simulink library "INT_InjSys_Co"  (R2016b)
settings: Solver=VariableStepAuto  StartTime=0.0  StopTime=10.0  RelTol=1e-3
settings Model: Creator=Administrator  LastModifiedBy=Administrator

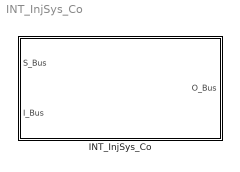
== system INT_InjSys_Co ==
  INT_InjSys_Co : Subsystem

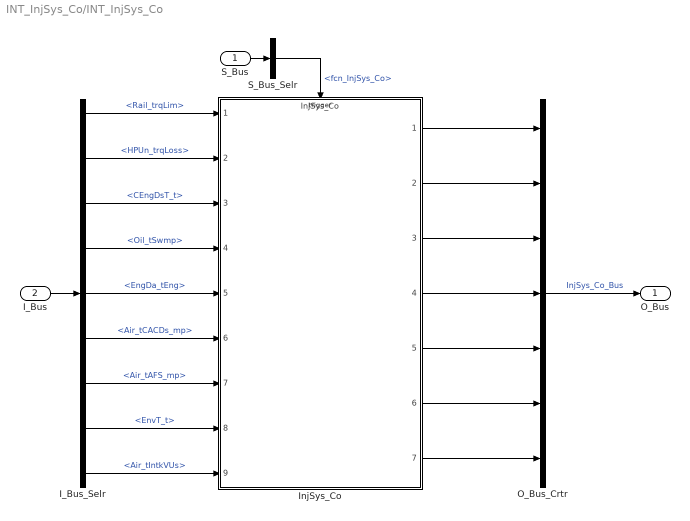
== system INT_InjSys_Co/INT_InjSys_Co ==
  S_Bus : Inport
  I_Bus : Inport  Port=2
  I_Bus_Selr : BusSelector  OutputSignals=Rail_trqLim,HPUn_trqLoss,CEngDsT_t,Oil_tSwmp,EngDa_tEng,Air_tCACDs_mp,Air_tAFS_mp,EnvT_t,Air_tIntkVUs
  InjSys_Co : ModelReference  ModelNameDialog=InjSys_Co  SimulationMode=Normal  ModelReferenceVersion=1.12  TriggerPortName=function  TriggerPortTriggerType=function-call  TriggerPortStatesWhenEnabling=held
  O_Bus_Crtr : BusCreator  Inputs=7
  S_Bus_Selr : BusSelector  OutputSignals=fcn_InjSys_Co
  O_Bus : Outport
  wires:
  S_Bus_Selr/1 -> InjSys_Co/Trigger  "<fcn_InjSys_Co>"
  S_Bus/1 -> S_Bus_Selr/1
  I_Bus/1 -> I_Bus_Selr/1
  I_Bus_Selr/1 -> InjSys_Co/1  "<Rail_trqLim>"
  I_Bus_Selr/2 -> InjSys_Co/2  "<HPUn_trqLoss>"
  I_Bus_Selr/3 -> InjSys_Co/3  "<CEngDsT_t>"
  I_Bus_Selr/4 -> InjSys_Co/4  "<Oil_tSwmp>"
  I_Bus_Selr/5 -> InjSys_Co/5  "<EngDa_tEng>"
  I_Bus_Selr/6 -> InjSys_Co/6  "<Air_tCACDs_mp>"
  I_Bus_Selr/7 -> InjSys_Co/7  "<Air_tAFS_mp>"
  I_Bus_Selr/8 -> InjSys_Co/8  "<EnvT_t>"
  I_Bus_Selr/9 -> InjSys_Co/9  "<Air_tIntkVUs>"
  O_Bus_Crtr/1 -> O_Bus/1  "InjSys_Co_Bus"
  InjSys_Co/1 -> O_Bus_Crtr/1
  InjSys_Co/2 -> O_Bus_Crtr/2
  InjSys_Co/3 -> O_Bus_Crtr/3
  InjSys_Co/4 -> O_Bus_Crtr/4
  InjSys_Co/5 -> O_Bus_Crtr/5
  InjSys_Co/6 -> O_Bus_Crtr/6
  InjSys_Co/7 -> O_Bus_Crtr/7
